simulink model "iss_sim"  (R2014a)
settings: Solver=ode45  StartTime=0.0  StopTime=10.0  RelTol=1e-3
values from neighbouring files (symbols this model uses):
  iss_sys = sys_class    [create_all_sys.m]
settings Model: Creator=UX31  LastModifiedBy=UX31

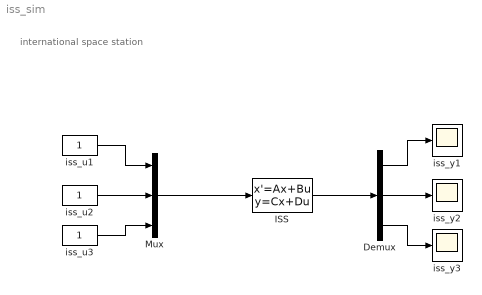
== system iss_sim ==
  note: international space station
  Demux : Demux  Outputs=3
  ISS : StateSpace  A=iss_sys.sys.a  B=iss_sys.sys.b  C=iss_sys.sys.c  D=iss_sys.sys.d  X0=iss_sys.x0_lb
  Mux : Mux  Inputs=3
  iss_u1 : Constant
  iss_u2 : Constant
  iss_u3 : Constant
  iss_y1 : Scope
  iss_y2 : Scope
  iss_y3 : Scope
      settings: SaveName=ScopeData2
  wires:
  Mux/1 -> ISS/1
  iss_u1/1 -> Mux/1
  iss_u2/1 -> Mux/2
  iss_u3/1 -> Mux/3
  ISS/1 -> Demux/1
  Demux/1 -> iss_y1/1
  Demux/2 -> iss_y2/1
  Demux/3 -> iss_y3/1
